simulink model "Smart_three_phase_APFC"  (R2024b)
settings: Solver=VariableStepAuto  StartTime=0.0  StopTime=50  RelTol=1e-3
libraries: spsThreePhaseSeriesRLCLoadLib x7, spsThreePhaseBreakerLib x7, dspstat3 x4, spsThreePhaseSourceLib x1, spsPowerLib x1, spsThreePhaseVIMeasurementLib x1, sps_lib x1
settings Model: Creator=shaunwin pereira  LastModifiedBy=shaunwin pereira

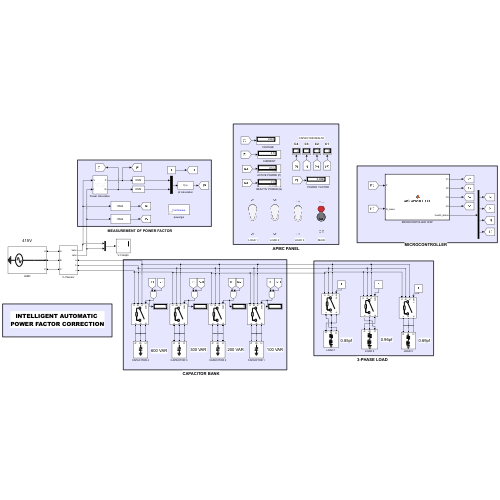
[thumbnail: Simulink's stored preview of the top-level diagram]
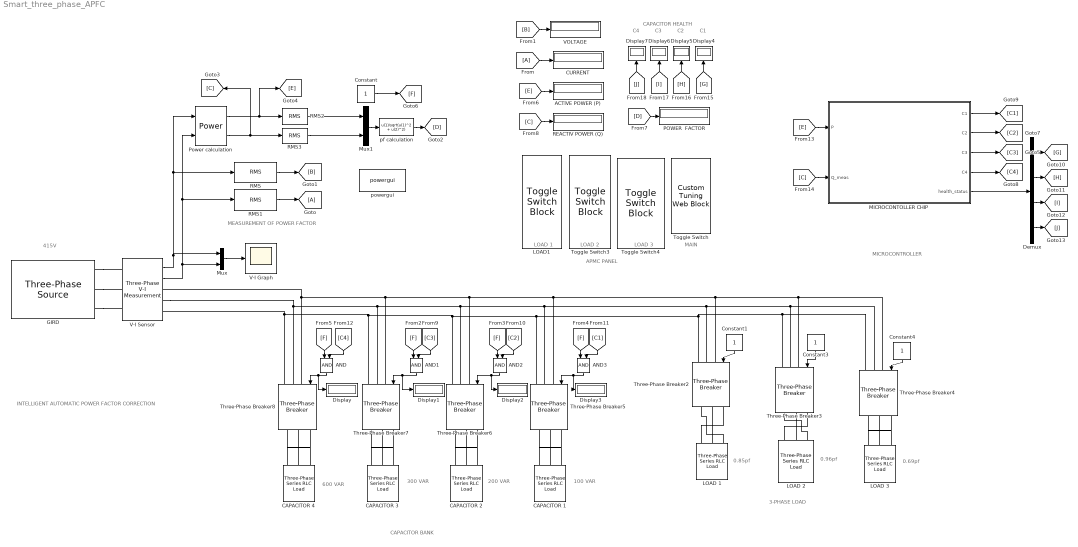
== system Smart_three_phase_APFC ==
  note: CAPACITOR HEALTH
  note: C1
  note: 0.69pf
  note: INTELLIGENT AUTOMATIC
      | POWER FACTOR CORRECTION
  note: APMC PANEL
  note: MAIN
  note: LOAD 1
  note: LOAD 2
  note: LOAD 3
  note: MEASUREMENT OF POWER FACTOR
  note: 3-PHASE LOAD
  note: CAPACITOR BANK
  note: MICROCONTROLLER
  note: 0.85pf
  note: 0.96pf
  note: 300 VAR
  note: 200 VAR
  note: 100 VAR
  note: 600 VAR
  note: 415V
  note: C2
  note: C3
  note: C4
  ACTIVE POWER (P) : Display
  AND{,1..3} (4 alike) : Logic  IconShape=distinctive  AllPortsSameDT=off  OutDataTypeStr=boolean
  CAPACITOR 1 : spsThreePhaseSeriesRLCLoadLib/Three-Phase Series RLC Load  LConnTagsString=A|B|C  Configuration=Y (grounded)  NominalVoltage=415  Vabc=[1e3 1e3 1e3]  Vabcp=[1e3 1e3 1e3]  NominalFrequency=50  UnbalancedPower=off  ActivePower=0  InductivePower=0  CapacitivePower=100  Pabc=[10e3 9e3 11e3]  QLabc=[100 90 110]  QCabc=[100 90 110]  Pabcp=[10e3 9e3 11e3]  QLabcp=[100 90 110]  QCabcp=[100 90 110]  Measurements=None  LoadType=constant Z
  CAPACITOR 2 : spsThreePhaseSeriesRLCLoadLib/Three-Phase Series RLC Load  LConnTagsString=A|B|C  Configuration=Y (grounded)  NominalVoltage=415  Vabc=[1e3 1e3 1e3]  Vabcp=[1e3 1e3 1e3]  NominalFrequency=50  UnbalancedPower=off  ActivePower=0  InductivePower=0  CapacitivePower=200  Pabc=[10e3 9e3 11e3]  QLabc=[100 90 110]  QCabc=[100 90 110]  Pabcp=[10e3 9e3 11e3]  QLabcp=[100 90 110]  QCabcp=[100 90 110]  Measurements=None  LoadType=constant Z
  CAPACITOR 3 : spsThreePhaseSeriesRLCLoadLib/Three-Phase Series RLC Load  LConnTagsString=A|B|C  Configuration=Y (grounded)  NominalVoltage=415  Vabc=[1e3 1e3 1e3]  Vabcp=[1e3 1e3 1e3]  NominalFrequency=50  UnbalancedPower=off  ActivePower=0  InductivePower=0  CapacitivePower=300  Pabc=[10e3 9e3 11e3]  QLabc=[100 90 110]  QCabc=[100 90 110]  Pabcp=[10e3 9e3 11e3]  QLabcp=[100 90 110]  QCabcp=[100 90 110]  Measurements=None  LoadType=constant Z
  CAPACITOR 4 : spsThreePhaseSeriesRLCLoadLib/Three-Phase Series RLC Load  LConnTagsString=A|B|C  Configuration=Y (grounded)  NominalVoltage=415  Vabc=[1e3 1e3 1e3]  Vabcp=[1e3 1e3 1e3]  NominalFrequency=50  UnbalancedPower=off  ActivePower=0  InductivePower=0  CapacitivePower=600  Pabc=[10e3 9e3 11e3]  QLabc=[100 90 110]  QCabc=[100 90 110]  Pabcp=[10e3 9e3 11e3]  QLabcp=[100 90 110]  QCabcp=[100 90 110]  Measurements=None  LoadType=constant Z
  CURRENT : Display
  Constant{,1,3..4} (4 alike) : Constant
  Demux : Demux
  Display{,1..7} (8 alike) : Display
  From : From
  GIRD : spsThreePhaseSourceLib/Three-Phase Source  InternalConnection=Yg  VoltagePhases=off  Voltage=415  PhaseAngle=0  Voltage_phases=[25e3 25e3 25e3]/sqrt(3)  PhaseAngles_phases=[0 -120 +120]  Frequency=50  NonIdealSource=on  SpecifyImpedance=off  Resistance=0  Inductance=0  ShortCircuitLevel=100e6  BaseVoltage=415  XRratio=7  BusType=swing  Pref=10e3  Qref=0  Prefabc=[10e3, 10e3, 10e3]  Qrefabc=[0, 0, 0]  Qmin=-inf  Qmax=inf
  Goto : Goto
  LOAD 1 : spsThreePhaseSeriesRLCLoadLib/Three-Phase Series RLC Load  LConnTagsString=A|B|C  Configuration=Y (grounded)  NominalVoltage=415  Vabc=[1e3 1e3 1e3]  Vabcp=[1e3 1e3 1e3]  NominalFrequency=50  UnbalancedPower=off  ActivePower=500  InductivePower=312  CapacitivePower=0  Pabc=[10e3 9e3 11e3]  QLabc=[100 90 110]  QCabc=[100 90 110]  Pabcp=[10e3 9e3 11e3]  QLabcp=[100 90 110]  QCabcp=[100 90 110]  Measurements=None  LoadType=constant Z
  LOAD 2 : spsThreePhaseSeriesRLCLoadLib/Three-Phase Series RLC Load  LConnTagsString=A|B|C  Configuration=Y (grounded)  NominalVoltage=415  Vabc=[1e3 1e3 1e3]  Vabcp=[1e3 1e3 1e3]  NominalFrequency=50  UnbalancedPower=off  ActivePower=1000  InductivePower=289  CapacitivePower=0  Pabc=[10e3 9e3 11e3]  QLabc=[100 90 110]  QCabc=[100 90 110]  Pabcp=[10e3 9e3 11e3]  QLabcp=[100 90 110]  QCabcp=[100 90 110]  Measurements=None  LoadType=constant Z
  LOAD 3 : spsThreePhaseSeriesRLCLoadLib/Three-Phase Series RLC Load  LConnTagsString=A|B|C  Configuration=Y (grounded)  NominalVoltage=415  Vabc=[1e3 1e3 1e3]  Vabcp=[1e3 1e3 1e3]  NominalFrequency=50  UnbalancedPower=off  ActivePower=1000  InductivePower=105  CapacitivePower=0  Pabc=[10e3 9e3 11e3]  QLabc=[100 90 110]  QCabc=[100 90 110]  Pabcp=[10e3 9e3 11e3]  QLabcp=[100 90 110]  QCabcp=[100 90 110]  Measurements=None  LoadType=constant Z
  LOAD1 : ToggleSwitchBlock  LabelPosition=Hide
      settings: Values={{'Off', 'On'}, [0 1]}
  MICROCONTOLLER CHIP : MATLAB Function  TreatAsAtomicUnit=on
  Mux : Mux  Inputs=2
  Mux1 : Mux  Inputs=2
  POWER  FACTOR : Display
  Power calculation : spsPowerLib/Power  Freq=50  Vinit=[1, 0]  Iinit=[1, 0]  Ts=0
  REACTIV POWER (Q) : Display
  RMS{,1..3} (4 alike) : dspstat3/RMS  run=off  directionMode=Each column  dimension=1  InputProcessing=Columns as channels (frame based)  reset_popup=None
  Three-Phase Breaker{2..8} (7 alike) : spsThreePhaseBreakerLib/Three-Phase Breaker  InitialState=open  SwitchA=on  SwitchB=on  SwitchC=on  SwitchTimes="[1/60  5/60]"  External=on  BreakerResistance=0.01  SnubberResistance=1e6  SnubberCapacitance=inf  Measurements=None
  Toggle Switch : CustomTuningWebBlock  LabelPosition=Hide  ShowInitialText=on  Configuration="{\"components\":[{\"name\":\"CustomSwitchStateComponent\",\"settings\":{\"position\":[0,0,1,1],\"showAllLabels\":1,\"states\":[{\"HitRegion\":{\"position\":[0.5,0,1,0.5]},\"Image\":{\"position\":[0,0.24928571428571428,0.5014285714285714,1],\"size\":[0.5014285714285714,1],\"src\":\"data:image\\/svg+xml;base64,PHN2ZyB4bWxucz0iaHR0cDovL3d3dy53My5vcmcvMjAwMC9zdmciIHhtbG5zOnhsaW5rPSJodHRwOi8vd3d3LnczLm9yZy8xOTk5L3hsaW5rIiB2aWV3Qm94PSIwIDAgMzguMDQgMTUwIj48ZGVmcz48c3R5bGU+LmNscy0xe2ZpbGw6dXJsKCNyYWRpYWwtZ3JhZGllbnQpO30uY2xzLTJ7ZmlsbDp1cmwoI3JhZGlhbC1ncmFkaWVudC0yKTt9LmNscy0ze2ZpbGw6dXJsKCNXaGl0ZV9CbGFjayk7fS5jbHMtNHtmaWxsOnVybCgjcmFkaWFsLWdyYWRpZW50LTMpO30uY2xzLTV7ZmlsbDojNWI1YjViO30uY2xzLTZ7ZmlsbDp1cmwoI3Jh ...(+3556 chars)\",\"srcOrientation\":\"Right\"},\"Label\":{\"color\":[0.5019607843137255,0.5019607843137255,0.5019607843137255],\"icon\":{\"size\":[0,0],\"src\":[],\"srcOrientation\":\"Right\"},\"iconOffset\":0,\"iconPlacement\":\"left\",\"opacity\":1,\"position\":[0.92,0.5],\"show\":true,\"text\":{\"content\":\"Off\",\"font\":\"Helvetica\"}},\"Value\":0},{\"HitRegion\":{\"position\":[0,0,1,0.5]},\"Image\":{\"position\":[0,0.24928571428571428,0.5014285714285714,1],\"size\":[0.5014285714285714,1],\"src\":\"data:image\\/svg+xml;base64,PHN2ZyB4bWxucz0iaHR0cDovL3d3dy53My5vcmcvMjAwMC9zdmciIHhtbG5zOnhsaW5rPSJodHRwOi8vd3d3LnczLm9yZy8xOTk5L3hsaW5rIiB2aWV3Qm94PSIwIDAgMzguMDQgMTUwIj48ZGVmcz48c3R5bGU+LmNscy0xe2ZpbGw6dXJsKCNyYWRpYWwtZ3JhZGllbnQpO30uY2xzLTJ7ZmlsbDp1cmwoI3JhZGlhbC1ncmFkaWVudC0yKTt9LmNscy0ze2ZpbGw6dXJsKCNXaGl0ZV9CbGFjayk7fS5jbHMtNHtmaWxsOnVybCgjcmFkaWFsLWdyYWRpZW50LTMpO30uY2xzLTV7ZmlsbDojNWI1YjViO30uY2xzLTZ7ZmlsbDp1cmwoI3Jh ...(+3628 chars)\",\"srcOrientation\":\"Right\"},\"Label\":{\"color\":[0.5019607843137255,0.5019607843137255,0.5019607843137255],\"icon\":{\"size\":[0,0],\"src\":[],\"srcOrientation\":\"Right\"},\"iconOffset\":0,\"iconPlacement\":\"left\",\"opacity\":1,\"position\":[0.08,0.5],\"show\":true,\"text\":{\"content\":\"On\",\"font\":\"Helvetica\"}},\"Value\":1}]}},{\"name\":\"BackgroundImageComponent\",\"settings\":{\"image\":{\"size\":[70,135],\"src\":\"default\",\"srcOrientation\":\"Right\"},\"position\":[0,0,1,1],\"scaleMode\":\"0\"}},{\"name\":\"ForegroundImageComponent\",\"settings\":{\"image\":{\"size\":[0,0],\"src\":\"default\",\"srcOrientation\":[]},\"isForeground\":1,\"position\":[0,0,1,1],\"scaleMode\":\"0\"}}],\"settings\":{\"BindingType\":\"param\",\"backgroundColor\":[0,0,0],\"backgroundOffset\":0.14,\"fixedAspectRatio\":\"on\",\"foregroundColor\":[0,0,0],\"showBackgroundColor\":false,\"variant\":\"toggle\",\"version\":\"R2024b\"},\"type\":\"Switch\"}"
  Toggle Switch3 : ToggleSwitchBlock  LabelPosition=Hide
      settings: Values={{'Off', 'On'}, [0 1]}
  Toggle Switch4 : ToggleSwitchBlock  LabelPosition=Hide
      settings: Values={{'Off', 'On'}, [0 1]}
  V-I Graph : Scope
  V-I Sensor : spsThreePhaseVIMeasurementLib/Three-Phase V-I Measurement  VoltageMeasurement=phase-to-ground  SetLabelV=off  LabelV=Vabc  Vpu=off  VpuLL=off  CurrentMeasurement=yes  SetLabelI=off  LabelI=Iabc  Ipu=off  Pbase=100e6  Vbase=500e3  OutputType=Complex  PhasorSimulation=off  PSBequivalent=0
  VOLTAGE : Display
  pf calculation : Fcn  Expr=u(1)/sqrt(u(1)^2 + u(2)^2)
  powergui : sps_lib/powergui  Priority=1  SimulationMode=Continuous  SampleTime=50e-6  frequency=60  Iterations=50  frequencyindice=50  Pbase=100e6  ErrMax=1e-4  UnitsV=kV  UnitsW=MW  buscounter=0  FunctionMessages=off  echomessages=off  EnableUseOfTLC=off  CurrentSourceSwitches=off  DisableSnubberDevices=off  DisableRonSwitches=off  DisableVfSwitches=off  DisplayEquations=off  AutomaticDiscreteSolvers=off  SolverType=Tustin/Backward Euler (TBE)  Interpol=off  ExternalGateDelay=off  methode=off  Ts=100  x0status=blocks  SPID=on  SwTol=0  HookPort=off  NonlinearTolerance=1e-4  nMaxIteration=100  ContinueOnMaxIteration=off  RestoreLinks=warning  ResistiveCurrentMeasurement=off  Frange=[0:2:500]  Ylog=off  Xlog=on  ShowGrid=off  save=off  variable=ZData  structure=0  ZoomFFT=off  StartTime=0.0  cycles=1  DisplayStyle=1  fundamental=60  FreqAxis=off  MaxFrequency=1000  frequencyindicesteady=1  RmsSteady=1  display=off
  wires:
  Constant1/1 -> Three-Phase Breaker2/1
  pf calculation/1 -> [D]
  Constant3/1 -> Three-Phase Breaker3/1
  Constant4/1 -> Three-Phase Breaker4/1
  AND3/1 -> Display3/1, Three-Phase Breaker5/1
  AND2/1 -> Display2/1, Three-Phase Breaker6/1
  AND1/1 -> Display1/1, Three-Phase Breaker7/1
  AND/1 -> Display/1, Three-Phase Breaker8/1
  From/1 -> CURRENT/1
  RMS1/1 -> Goto/1
  RMS/1 -> [B]
  [B] -> VOLTAGE/1
  Mux/1 -> V-I Graph/1
  Mux1/1 -> pf calculation/1
  RMS3/1 -> Mux1/2
  RMS2/1 -> Mux1/1
  [F] -> AND/1
  [F] -> AND1/1
  [F] -> AND2/1
  [F] -> AND3/1
  [C4] -> AND/2
  [C3] -> AND1/2
  [C2] -> AND2/2
  [C1] -> AND3/2
  Power calculation/2 -> [C], RMS3/1
  V-I Sensor/1 -> Power calculation/1, RMS/1, Mux/1
  Power calculation/1 -> RMS2/1, [E]
  V-I Sensor/2 -> Power calculation/2, RMS1/1, Mux/2
  [C] -> REACTIV POWER (Q)/1
  [E] -> ACTIVE POWER (P)/1
  [D] -> POWER  FACTOR/1
  Constant/1 -> [F]
  [E] -> MICROCONTOLLER CHIP/1(P)
  [C] -> MICROCONTOLLER CHIP/2(Q_meas)
  MICROCONTOLLER CHIP/1(C1) -> [C1]
  MICROCONTOLLER CHIP/2(C2) -> [C2]
  MICROCONTOLLER CHIP/3(C3) -> [C3]
  MICROCONTOLLER CHIP/4(C4) -> [C4]
  MICROCONTOLLER CHIP/5(health_status) -> Demux/1
  Demux/1 -> [G]
  Demux/2 -> [H]
  Demux/3 -> [I]
  Demux/4 -> [J]
  [G] -> Display4/1
  [H] -> Display5/1
  [I] -> Display6/1
  [J] -> Display7/1
  connections:
  GIRD/RConn1 -- V-I Sensor/LConn1
  GIRD/RConn2 -- V-I Sensor/LConn2
  GIRD/RConn3 -- V-I Sensor/LConn3
  V-I Sensor/RConn2 -- Three-Phase Breaker7/LConn2 -- Three-Phase Breaker6/LConn2 -- Three-Phase Breaker4/LConn2 -- Three-Phase Breaker3/LConn2 -- Three-Phase Breaker2/LConn2 -- Three-Phase Breaker5/LConn2 -- Three-Phase Breaker8/LConn2
  Three-Phase Breaker2/LConn1 -- Three-Phase Breaker4/LConn1 -- Three-Phase Breaker3/LConn1 -- Three-Phase Breaker6/LConn1 -- Three-Phase Breaker7/LConn1 -- V-I Sensor/RConn1 -- Three-Phase Breaker8/LConn1 -- Three-Phase Breaker5/LConn1
  LOAD 1/LConn3 -- Three-Phase Breaker2/RConn3
  LOAD 1/LConn1 -- Three-Phase Breaker2/RConn1
  LOAD 1/LConn2 -- Three-Phase Breaker2/RConn2
  LOAD 2/LConn1 -- Three-Phase Breaker3/RConn1
  LOAD 2/LConn3 -- Three-Phase Breaker3/RConn3
  LOAD 2/LConn2 -- Three-Phase Breaker3/RConn2
  LOAD 3/LConn2 -- Three-Phase Breaker4/RConn2
  LOAD 3/LConn1 -- Three-Phase Breaker4/RConn1
  LOAD 3/LConn3 -- Three-Phase Breaker4/RConn3
  Three-Phase Breaker2/LConn3 -- Three-Phase Breaker3/LConn3 -- Three-Phase Breaker4/LConn3 -- Three-Phase Breaker5/LConn3 -- Three-Phase Breaker6/LConn3 -- Three-Phase Breaker7/LConn3 -- Three-Phase Breaker8/LConn3 -- V-I Sensor/RConn3
  CAPACITOR 1/LConn1 -- Three-Phase Breaker5/RConn1
  CAPACITOR 1/LConn3 -- Three-Phase Breaker5/RConn3
  CAPACITOR 1/LConn2 -- Three-Phase Breaker5/RConn2
  CAPACITOR 2/LConn3 -- Three-Phase Breaker6/RConn3
  CAPACITOR 2/LConn2 -- Three-Phase Breaker6/RConn2
  CAPACITOR 2/LConn1 -- Three-Phase Breaker6/RConn1
  CAPACITOR 3/LConn1 -- Three-Phase Breaker7/RConn1
  CAPACITOR 3/LConn2 -- Three-Phase Breaker7/RConn2
  CAPACITOR 3/LConn3 -- Three-Phase Breaker7/RConn3
  CAPACITOR 4/LConn2 -- Three-Phase Breaker8/RConn2
  CAPACITOR 4/LConn1 -- Three-Phase Breaker8/RConn1
  CAPACITOR 4/LConn3 -- Three-Phase Breaker8/RConn3

== matlab function Smart_three_phase_APFC/MICROCONTOLLER CHIP ==
  settings: updateMethod=DISCRETE
  data: P input; C1 output; Q_meas input; C2 output; C3 output; C4 output; health_status output
function [C1, C2, C3, C4, health_status] = apfc_advanced_logic(P, Q_meas)
    % 1. Memory and Health Initialization
    persistent caps_state;
    persistent timer;
    persistent cycle_counts; 
    
    if isempty(caps_state)
        caps_state = [0, 0, 0, 0];
        timer = 0; 
        cycle_counts = [0, 0, 0, 0];
    end
    
    timer = timer + 1;
    
    % Sum the inputs [Phase A; Phase B; Phase C] arrays
    P_total = sum(P);
    Q_total = sum(Q_meas);
    
    % 2. Health Monitoring Logic
    MAX_CYCLES = 10; 
    health_status = [0, 0, 0, 0]; 
    for i = 1:4
        if cycle_counts(i) > MAX_CYCLES
            health_status(i) = 1; % 1 = Degraded/Maintenance Required
        end
    end
    
    % 3. Safety Deadband (System OFF)
    if abs(P_total) < 20
        cycle_counts = cycle_counts + caps_state; 
        caps_state = [0, 0, 0, 0];
        C1 = 0; C2 = 0; C3 = 0; C4 = 0;
        return;
    end
    
    % 4. Main Control Logic execution every 500 steps
    if timer > 50
        timer = 0; 
        
        caps = [100, 200, 300, 600];
        Q_supplied = sum(caps_state .* caps);
        Q_true = Q_total + Q_supplied;
        
        % Calculate the exact error of our CURRENT state
        current_q_rem = Q_true - Q_supplied;
        current_cost = abs(current_q_rem);
        if current_q_rem < 0
            current_cost = current_cost * 1.5; 
        end
        
        % 5. Combinatorial Optimization & Priority Switching
        best_cost = inf;
        best_candidate = caps_state;
        
        % Test all 16 possible capacitor combinations
        for i = 0:15
            bits = bitget(i, 4:-1:1);
            q_cap = sum(bits .* caps);
            
            % Base Error Cost
            q_rem = Q_true - q_cap;
            cost = abs(q_rem);
            
            % Overcompensation Penalty
            if q_rem < 0
                cost = cost * 1.5;
            end
            
            % PRIORITY / HEALTH PENALTY
            wear_penalty = sum(bits .* (health_status * 200)); 
            cost = cost + wear_penalty;
            
            % SWITCHING PENALTY (Minimize total state transitions)
            transitions = sum(abs(bits - caps_state));
            switching_penalty = transitions * 10; 
            cost = cost + switching_penalty;
            
            % Save the lowest cost combination
            if cost < best_cost
                best_cost = cost;
                best_candidate = bits;
            end
        end
        
        % 6. Anti-Chattering Hysteresis
        hysteresis_band = 40; 
        if (current_cost - best_cost) > hysteresis_band
            state_changes = abs(best_candidate - caps_state);
            cycle_counts = cycle_counts + state_changes;
            caps_state = best_candidate;
        end
    end
    
    % 7. Assign Outputs
    C1 = caps_state(1);
    C2 = caps_state(2);
    C3 = caps_state(3);
    C4 = caps_state(4);
end
